simulink model "hcu_main_ADASwEPS"  (Simulink 8.2)
settings: Solver=FixedStepDiscrete  StartTime=0.0  StopTime=inf  FixedStep=0.001  RelTol=1e-3
PostLoadFcn:
  | , if any(exist('dsrtsu_mdlpostloadfcn', 'file') == [2, 3, 6]), try dsrtsu_mdlpostloadfcn('Execute', bdroot); catch fprintf('Error in PostLoadFcn (dsrtsu_mdlpostloadfcn) for model "%s":\n %s\n', bdroot, lasterr); end, end,
values from neighbouring files (symbols this model uses):
  C_TASK_1MS_S = (	C_TICK_TIME_S       )    [hcu_local_hdr.m]    (also in temp_ovrd_values.m = double(	0.001                  ))
  C_TASK_5MS_S = (	C_TICK_TIME_S      	)    [hcu_local_hdr.m]
  ENUM_ADASLFCSTATUS_OFF = uint8(  0  )    [hcu_local_hdr.m]
  ENUM_ADASLFCSTATUS_STANDBY = uint8(  1  )    [hcu_local_hdr.m]
  ENUM_ADASLKASTATUS_ACTIVE = uint8(  2  )    [hcu_local_hdr.m]
  ENUM_ADASLKASTATUS_OFF = uint8(  0  )    [hcu_local_hdr.m]
  ENUM_ADASLKASTATUS_STANDBY = uint8(  1  )    [hcu_local_hdr.m]
  ENUM_EPSMODEREQ_ANGLE = uint8(  1  )    [hcu_local_hdr.m]
  ENUM_EPSMODEREQ_INTERNAL = uint8(  0  )    [hcu_local_hdr.m]
  ENUM_EPSMODEREQ_TORQUE = uint8(  2  )    [hcu_local_hdr.m]
  ENUM_GEARPOSN_1ST = uint8(  1  )    [hcu_local_hdr.m]
  ENUM_GEARPOSN_2ND = uint8(  2  )    [hcu_local_hdr.m]
  ENUM_GEARPOSN_3RD = uint8(  3  )    [hcu_local_hdr.m]
  ENUM_GEARPOSN_4TH = uint8(  4  )    [hcu_local_hdr.m]
  ENUM_GEARPOSN_5TH = uint8(  5  )    [hcu_local_hdr.m]
  ENUM_GEARPOSN_6TH = uint8(  6  )    [hcu_local_hdr.m]
  ENUM_GEARPOSN_PN = uint8(  0  )    [hcu_local_hdr.m]
  ENUM_GEARPOSN_R = uint8(  7  )    [hcu_local_hdr.m]
  FALSE = boolean( 0 )    [hcu_local_hdr.m]
  TRUE = boolean( 1 )    [hcu_local_hdr.m]
undefined symbols (not defined in the file or in its folder): AACC_DistCtrlIMult_X_mps2, AACC_DistCtrlPMult_X_mps2, AACC_GearActual_enum, AACC_SpdCtrlIMult_X_mps2, AACC_SpdCtrlPMult_X_mps2, AACC_VehSpd_kph, AISP_EPSCurrent_pct, AISP_TqASensorDelta_pct, AISP_TqBSensorDelta_pct, ENUM_ACCSTATUS_ACTIVE, ENUM_ACCSTATUS_OFF, ENUM_ACCSTATUS_STANDBY, ENUM_ADASLFCSTATUS_ACTIVE, ENUM_ADASLFCSTATUS_TRANSITION, ENUM_LFCCCONTSTATUS_ACTIVE, ENUM_LFCCCONTSTATUS_NOTAVAIL_TEMP, ENUM_LFCCCONTSTATUS_OFF, ENUM_LFCCCONTSTATUS_READY, ENUM_LFCCCONTSTATUS_TRANSITION, ENUM_LKACCONTSTATUS_ACTIVE, ENUM_LKACCONTSTATUS_NOTAVAIL_TEMP, ENUM_LKACCONTSTATUS_OFF, ENUM_LKACCONTSTATUS_READY, KACC_AcclReqMax_g, KACC_AcclReqMin_g, KACC_ACCSetTimeGapDef1_s, KACC_ACCSetTimeGapDef2_s, KACC_ACCSetTimeGapDef3_s, KACC_ACCSetTimeGapDef4_s, KACC_ACCSetTimeGapDef5_s, KACC_AirDensity_kgpm3, KACC_AirDragCoef_rat, KACC_CommandsOn_flg, KACC_CruzSpdChgTimeThres_s, KACC_DecReqSwOffThres_Nm, KACC_DecReqSwOnThres_Nm, KACC_DistCtrlAdjTime_s, KACC_DistCtrlCalRate_s, KACC_DistCtrlIC_mps2, KACC_DistCtrlIGain_rat, KACC_DistCtrlIMax_mps2, KACC_DistCtrlIMin_mps2, KACC_DistCtrlIRest_flg, KACC_DistCtrlKGain_rat, KACC_DistCtrlPause_flg, KACC_DistCtrlPGain_rat, KACC_FinalDriveEff_pct, KACC_FinalDriveRatio_rat, KACC_FrontalArea_m2, KACC_GearBoxEff_pct, KACC_LongPushSpdChg_kph, KACC_MaxAccSetSpd_kph, KACC_MinAccSetSpd_kph, KACC_SetAllowSpdLim_kph, KACC_SpdCtrlAdjTime_s, KACC_SpdCtrlCalRate_s, KACC_SpdCtrlIC_mps2, KACC_SpdCtrlIGain_rat, KACC_SpdCtrlIMax_mps2, KACC_SpdCtrlIMin_mps2 ... (+26)
libraries: simulink x54, adas_lib x6, rti1401lib_dio_type3 x4, rtimmsu_dsrtlib x3, hcu_lib x2, aeb x1, ddm x1, dfr x1, dgi x1, dhp x1, dinr x1, dip x1
(part 7 of 9)

== system hcu_main_ADASwEPS/EPSS/EPSS/TorqueMode ==
  VISP_StrTqReq_Nm : Inport
  VISP_StrTqReqAppl_flg : Inport  Port=2
  VEPSS_StrWhlTqReqAst_Nm : Inport  Port=3
  VISP_EPSModeReq_enum : Inport  Port=4
  VISP_ADASLFCStatus_enum : Inport  Port=5
  VISP_ADASLFCMode_enum : Inport  Port=6
  Constant1 : Constant  Value=ENUM_LFCCCONTSTATUS_ACTIVE
  Constant10 : Constant  Value=ENUM_ADASLFCSTATUS_OFF
  Constant11 : Constant  Value=ENUM_LFCCCONTSTATUS_NOTAVAIL_TEMP
  Constant2 : Constant  Value=ENUM_LFCCCONTSTATUS_TRANSITION
  Constant3 : Constant  Value=ENUM_LFCCCONTSTATUS_READY
  Constant4 : Constant  Value=ENUM_ADASLFCSTATUS_TRANSITION
  Constant5 : Constant  Value=ENUM_LFCCCONTSTATUS_TRANSITION
  Constant6 : Constant  Value=ENUM_EPSMODEREQ_TORQUE
  Constant7 : Constant  Value=ENUM_ADASLFCSTATUS_ACTIVE
  Constant8 : Constant  Value=ENUM_LFCCCONTSTATUS_OFF
  Constant9 : Constant  Value=ENUM_ADASLFCSTATUS_STANDBY
  Logical Operator : Logic  Inputs=3  AllPortsSameDT=off  OutDataTypeStr=boolean
  Relational Operator{1..6} (6 alike) : RelationalOperator  Operator===  OutDataTypeStr=boolean
  Sum : Sum
  Switch{1..6} (6 alike) : Switch  Criteria=u2 ~= 0
  VEPSS_StrWhlTqReqTq_Nm : Outport
  VEPSS_TorqueModeActive_flg : Outport  Port=2
  VEPSS_LFCContStatusTq_enum : Outport  Port=3
  wires:
  Sum/1 -> Switch2/1
  VISP_StrTqReq_Nm/1 -> Switch2/3, Sum/2
  Switch4/1 -> VEPSS_StrWhlTqReqTq_Nm/1  "VEPSS_StrWhlTqReqTq_Nm"
  Constant1/1 -> Switch3/3
  Switch1/1 -> VEPSS_LFCContStatusTq_enum/1, [VEPSS_LFCContStatus_enum]  "VEPSS_LFCContStatusTq_enum"
  VEPSS_StrWhlTqReqAst_Nm/1 -> [VEPSS_StrWhlTqReqAst_Nm], Sum/1
  Switch2/1 -> Switch4/1
  VISP_ADASLFCMode_enum/1 -> Relational Operator1/1
  Constant4/1 -> Relational Operator1/2
  Switch3/1 -> Switch1/1
  Relational Operator1/1 -> Switch3/2
  Constant2/1 -> Switch3/1
  [VEPSS_TorqueModeActive_flg] -> Switch4/2
  [VEPSS_LFCContStatus_enum] -> Relational Operator2/1
  Constant5/1 -> Relational Operator2/2
  Relational Operator2/1 -> Switch2/2
  [VEPSS_StrWhlTqReqAst_Nm] -> Switch4/3
  [VEPSS_TorqueModeActive_flg] -> VEPSS_TorqueModeActive_flg/1  "VEPSS_TorqueModeActive_flg"
  VISP_EPSModeReq_enum/1 -> Relational Operator3/1
  Constant6/1 -> Relational Operator3/2
  VISP_StrTqReqAppl_flg/1 -> Logical Operator/1
  Logical Operator/1 -> Switch1/2, [VEPSS_TorqueModeActive_flg]
  Relational Operator3/1 -> Logical Operator/2
  Constant7/1 -> Relational Operator4/2
  Relational Operator4/1 -> Logical Operator/3
  Switch5/1 -> Switch1/3
  Constant9/1 -> Relational Operator5/2
  Relational Operator5/1 -> Switch5/2
  Constant3/1 -> Switch5/1
  Switch6/1 -> Switch5/3
  VISP_ADASLFCStatus_enum/1 -> Relational Operator6/1, Relational Operator5/1, Relational Operator4/1
  Constant10/1 -> Relational Operator6/2
  Relational Operator6/1 -> Switch6/2
  Constant8/1 -> Switch6/1
  Constant11/1 -> Switch6/3

== system hcu_main_ADASwEPS/EPSS/model_info/EmptySubsystem ==

== system hcu_main_ADASwEPS/ISP/AngleProcessing/Timer ==
  Enable : EnablePort  StatesWhenEnabling=reset
  C_TASK_1MS_S : Constant  Value=C_TASK_1MS_S
  Sum : Sum  Inputs=|++
  Unit Delay : UnitDelay  SampleTime=-1
  Unit Delay1 : UnitDelay  SampleTime=-1
  Time_s : Outport  OutputWhenDisabled=reset  InitialOutput=[0]
  wires:
  C_TASK_1MS_S/1 -> Unit Delay1/1
  Sum/1 -> Unit Delay/1, Time_s/1  "Time_s"
  Unit Delay/1 -> Sum/2
  Unit Delay1/1 -> Sum/1

== system hcu_main_ADASwEPS/ISP/AngleProcessing/Triggered Absolute Angle Zero ==
  In : Inport
  Trigger : TriggerPort
  SteerAngValid_flg : Constant  Value=TRUE
  Out1 : Outport
  Out2 : Outport  Port=2
  wires:
  In/1 -> Out1/1
  SteerAngValid_flg/1 -> Out2/1

== system hcu_main_ADASwEPS/ISP/PassThrough/EPSDegTest ==
  PassThrough : Inport
  AmplitudeDeg_pct : Constant  Value=5
  Compare To Constant : simulink/Logic and Bit Operations/Compare To Constant  relop===  const=3.0  OutDataTypeStr=boolean
  Constant : Constant  Value=2*pi  OutDataTypeStr=single
  DegSetPt : Constant
  FrequencyDeg_Hz : Constant
  Multiport Switch1 : MultiPortSwitch  Inputs=4
  Product : Product  Inputs=3  RndMeth=Zero
  Product1 : Product  RndMeth=Zero
  TestModeDeg_Sw : Constant
  Timer : Subsystem
  Trigonometric Funcon : Trigonometry
  DegOut : Outport
  wires:
  Multiport Switch1/1 -> DegOut/1  "DegOut"
  PassThrough/1 -> Multiport Switch1/2
  DegSetPt/1 -> Multiport Switch1/3
  Product1/1 -> Multiport Switch1/4
  FrequencyDeg_Hz/1 -> Product/2
  Product/1 -> Trigonometric Funcon/1
  AmplitudeDeg_pct/1 -> Product1/2
  Trigonometric Funcon/1 -> Product1/1
  Constant/1 -> Product/3
  Timer/1(SineTime_s) -> Product/1
  TestModeDeg_Sw/1 -> Compare To Constant/1, Multiport Switch1/1
  Compare To Constant/1 -> Timer/Enable

== system hcu_main_ADASwEPS/ISP/TqProcessing/LowPassFilter ==
  Raw : Inport
  Constant1 : Constant  OutDataTypeStr=single  SampleTime=-1
  LowPassCoef : Constant  SampleTime=-1
  Product : Product  RndMeth=Zero
  Product1 : Product  RndMeth=Zero
  Sum1 : Sum  Inputs=+-
  Sum2 : Sum
  Unit Delay1 : UnitDelay  SampleTime=-1
  Out : Outport
  wires:
  Raw/1 -> Product/2
  Constant1/1 -> Sum1/1
  LowPassCoef/1 -> [LowPassCoef], Product/1
  [LowPassCoef] -> Sum1/2
  Unit Delay1/1 -> Product1/1
  Sum1/1 -> Product1/2
  Product/1 -> Sum2/1
  Product1/1 -> Sum2/2
  Sum2/1 -> Unit Delay1/1, Out/1

== system hcu_main_ADASwEPS/ISP/TqProcessing/TorqueValid ==
  TqA : Inport
  TqB : Inport  Port=2
  Abs1 : Abs
  FALSE : Constant  Value=FALSE  OutDataTypeStr=single  SampleTime=-1
  Relational Operator1 : RelationalOperator  Operator=<=  OutDataTypeStr=boolean
  Sum1 : Sum  Inputs=+-
  Switch1 : Switch  Criteria=u2 ~= 0
  TRUE : Constant  Value=TRUE  OutDataTypeStr=single  SampleTime=-1
  TqValidThres_Nm : Constant  OutDataTypeStr=single  SampleTime=-1
  TqValid_flg : Outport
  wires:
  TRUE/1 -> Switch1/1
  TqValidThres_Nm/1 -> Relational Operator1/2
  Relational Operator1/1 -> Switch1/2
  Sum1/1 -> Abs1/1
  Abs1/1 -> Relational Operator1/1
  FALSE/1 -> Switch1/3
  Switch1/1 -> TqValid_flg/1  "TqValid_flg"
  TqA/1 -> Sum1/1
  TqB/1 -> Sum1/2

== system hcu_main_ADASwEPS/ISP/TqProcessing/TqSensorAZero ==
  VHAL_TqSensorADuty_pct : Inport
  TqSensorFlac_pct : Inport  Port=2
  KISP_EPSZeroReset_flg : Inport  Port=3
  Constant1 : Constant  Value=60  OutDataTypeStr=single  SampleTime=-1
  Constant2 : Constant  Value=50  OutDataTypeStr=single  SampleTime=-1
  Delay : Delay  DelayLength=1  InitialCondition=0
  Delay1 : Delay  DelayLength=1  InitialCondition=1
  Delay2 : Delay  DelayLength=1  InitialCondition=1
  FALSE : Constant  Value=FALSE
  Gain : Gain  Gain=-1
  IsInRange : adas_lib/IsInRange
  IsInRange1 : adas_lib/IsInRange
  KISP_CheckZeroTime_s : Constant  Value=3
  Latch : Subsystem
  Logical Operator : Logic  Operator=NOT  AllPortsSameDT=off  OutDataTypeStr=boolean
  Logical Operator1 : Logic  Operator=OR  AllPortsSameDT=off  OutDataTypeStr=boolean
  Logical Operator4 : Logic  AllPortsSameDT=off  OutDataTypeStr=boolean
  Relational Operator : RelationalOperator  Operator=<=  OutDataTypeStr=boolean
  Subtract : Sum  Inputs=+-
  Subtract1 : Sum  Inputs=+-
  Switch : Switch  Criteria=u2 ~= 0
  Switch1 : Switch  Criteria=u2 ~= 0
  Timer : Subsystem
  zero : Outport
  delta : Outport  Port=2
  wires:
  Relational Operator/1 -> Switch/2
  Logical Operator1/1 -> Latch/2(update)
  KISP_EPSZeroReset_flg/1 -> Logical Operator1/1
  Delay1/1 -> Logical Operator1/2
  Latch/1(out) -> Subtract/2, Switch/3
  Switch/1 -> Delay/1, Subtract1/2, zero/1
  KISP_CheckZeroTime_s/1 -> Relational Operator/2
  Timer/1(Time_s) -> Relational Operator/1
  Subtract/1 -> IsInRange/1
  VHAL_TqSensorADuty_pct/1 -> Subtract/1, IsInRange1/1, Switch1/1, Subtract1/1, Latch/1(in)
  Gain/1 -> IsInRange/3
  TqSensorFlac_pct/1 -> Gain/1, IsInRange/2
  Subtract1/1 -> delta/1
  IsInRange/1 -> Logical Operator4/2, Logical Operator/1
  Switch1/1 -> Switch/1
  Logical Operator/1 -> Delay1/1
  FALSE/1 -> Delay2/1
  Delay2/1 -> Switch1/2
  Delay/1 -> Switch1/3
  Logical Operator4/1 -> Timer/Enable
  IsInRange1/1 -> Logical Operator4/1
  Constant1/1 -> IsInRange1/2
  Constant2/1 -> IsInRange1/3

== system hcu_main_ADASwEPS/ISP/TqProcessing/TqSensorBZero ==
  VHAL_TqSensorBDuty_pct : Inport
  TqSensorFlac_pct : Inport  Port=2
  KISP_EPSZeroReset_flg : Inport  Port=3
  Constant1 : Constant  Value=60  OutDataTypeStr=single  SampleTime=-1
  Constant2 : Constant  Value=50  OutDataTypeStr=single  SampleTime=-1
  Delay : Delay  DelayLength=1  InitialCondition=0
  Delay1 : Delay  DelayLength=1  InitialCondition=1
  Delay2 : Delay  DelayLength=1  InitialCondition=1
  FALSE : Constant  Value=FALSE
  Gain : Gain  Gain=-1
  IsInRange : adas_lib/IsInRange
  IsInRange1 : adas_lib/IsInRange
  KISP_CheckZeroTime_s : Constant  Value=3
  Latch : Subsystem
  Logical Operator : Logic  Operator=NOT  AllPortsSameDT=off  OutDataTypeStr=boolean
  Logical Operator1 : Logic  Operator=OR  AllPortsSameDT=off  OutDataTypeStr=boolean
  Logical Operator4 : Logic  AllPortsSameDT=off  OutDataTypeStr=boolean
  Relational Operator : RelationalOperator  Operator=<=  OutDataTypeStr=boolean
  Subtract : Sum  Inputs=+-
  Subtract1 : Sum  Inputs=+-
  Switch : Switch  Criteria=u2 ~= 0
  Switch1 : Switch  Criteria=u2 ~= 0
  Timer : Subsystem
  zero : Outport
  delta : Outport  Port=2
  wires:
  Constant2/1 -> IsInRange1/3
  Constant1/1 -> IsInRange1/2
  IsInRange1/1 -> Logical Operator4/1
  Logical Operator4/1 -> Timer/Enable
  Delay/1 -> Switch1/3
  Delay2/1 -> Switch1/2
  FALSE/1 -> Delay2/1
  Logical Operator/1 -> Delay1/1
  Switch1/1 -> Switch/1
  IsInRange/1 -> Logical Operator/1, Logical Operator4/2
  Subtract1/1 -> delta/1
  TqSensorFlac_pct/1 -> IsInRange/2, Gain/1
  Gain/1 -> IsInRange/3
  VHAL_TqSensorBDuty_pct/1 -> Subtract/1, IsInRange1/1, Subtract1/1, Switch1/1, Latch/1(in)
  Subtract/1 -> IsInRange/1
  Timer/1(Time_s) -> Relational Operator/1
  KISP_CheckZeroTime_s/1 -> Relational Operator/2
  Switch/1 -> zero/1, Subtract1/2, Delay/1
  Latch/1(out) -> Switch/3, Subtract/2
  Delay1/1 -> Logical Operator1/2
  KISP_EPSZeroReset_flg/1 -> Logical Operator1/1
  Logical Operator1/1 -> Latch/2(update)
  Relational Operator/1 -> Switch/2

== system hcu_main_ADASwEPS/OSP/OSP/CheckSum Calculation ==
  BISP_outputs : Inport
  LifeCount : Inport  Port=2
  Byte0 : Subsystem
  Byte1 : Subsystem
  Byte2 : Subsystem
  Byte3 : Subsystem
  ChecksumCalculation : Subsystem  TreatAsAtomicUnit=on
  VOSP_SAS1CalcChecksum_raw8 : Outport
  wires:
  Byte0/2(ForByte1) -> Byte1/1(ForByte1)
  BISP_outputs/1 -> Byte0/1(BISP_outputs), Byte3/1(BISP_outputs)
  LifeCount/1 -> ChecksumCalculation/5(SAS_MsgCount)
  ChecksumCalculation/1(Message_Checksum) -> VOSP_SAS1CalcChecksum_raw8/1  "VOSP_SAS1CalcChecksum_raw8"
  Byte0/1(Byte0) -> ChecksumCalculation/1(Byte0)
  Byte1/1(Byte1) -> ChecksumCalculation/2(Byte1)
  Byte3/1(Byte3) -> ChecksumCalculation/4(Byte3)
  Byte2/1(Byte2) -> ChecksumCalculation/3(Byte2)

== system hcu_main_ADASwEPS/OSP/OSP/CheckSum Calculation1 ==
  BISP_outputs : Inport
  LifeCount : Inport  Port=2
  Byte0 : Subsystem
  Byte1 : Subsystem
  Byte2 : Subsystem
  Byte3 : Subsystem
  ChecksumCalculation : Subsystem  TreatAsAtomicUnit=on
  Terminator : Terminator
  VOSP_EPAS2CalcChecksum_raw8 : Outport
  wires:
  ChecksumCalculation/1(Message_Checksum) -> VOSP_EPAS2CalcChecksum_raw8/1  "VOSP_EPAS2CalcChecksum_raw8"
  LifeCount/1 -> ChecksumCalculation/5(EPAS2_MsgCount)
  BISP_outputs/1 -> Byte2/1(BISP_outputs), Byte3/1(BISP_outputs), Byte1/1(BISP_outputs)
  Byte0/1(Byte0) -> ChecksumCalculation/1(Byte0)
  Byte1/1(Byte1) -> ChecksumCalculation/2(Byte1)
  Byte2/1(Byte2) -> ChecksumCalculation/3(Byte2)
  Byte3/1(Byte3) -> ChecksumCalculation/4(Byte3)
  Byte3/2(ForByte4) -> Terminator/1

== system hcu_main_ADASwEPS/OSP/OSP/RollCnt ==
  max : Inport
  Add : Sum
  Constant : Constant  OutDataTypeStr=Inherit: Inherit via back propagation
  Constant1 : Constant  Value=0  OutDataTypeStr=Inherit: Inherit via back propagation
  Data Type Conversion6 : DataTypeConversion  OutDataTypeStr=uint8
  Relational Operator : RelationalOperator  Operator=>  OutDataTypeStr=boolean
  Switch2 : Switch  Criteria=u2 ~= 0
  Unit Delay1 : UnitDelay  SampleTime=-1
  out : Outport
  wires:
  Constant/1 -> Add/1
  Add/1 -> Switch2/3, Relational Operator/1
  Unit Delay1/1 -> Add/2
  Constant1/1 -> Switch2/1
  Switch2/1 -> Unit Delay1/1, Data Type Conversion6/1
  max/1 -> Relational Operator/2
  Relational Operator/1 -> Switch2/2
  Data Type Conversion6/1 -> out/1

== system hcu_main_ADASwEPS/OSP/OSP/RollCnt1 ==
  max : Inport
  Add : Sum
  Constant : Constant  OutDataTypeStr=Inherit: Inherit via back propagation
  Constant1 : Constant  Value=0  OutDataTypeStr=Inherit: Inherit via back propagation
  Data Type Conversion6 : DataTypeConversion  OutDataTypeStr=uint8
  Relational Operator : RelationalOperator  Operator=>  OutDataTypeStr=boolean
  Switch2 : Switch  Criteria=u2 ~= 0
  Unit Delay1 : UnitDelay  SampleTime=-1
  out : Outport
  wires:
  Data Type Conversion6/1 -> out/1
  Relational Operator/1 -> Switch2/2
  max/1 -> Relational Operator/2
  Switch2/1 -> Data Type Conversion6/1, Unit Delay1/1
  Constant1/1 -> Switch2/1
  Unit Delay1/1 -> Add/2
  Add/1 -> Relational Operator/1, Switch2/3
  Constant/1 -> Add/1

== system hcu_main_ADASwEPS/OSP/OSP/RollCnt2 ==
  max : Inport
  Add : Sum
  Constant : Constant  OutDataTypeStr=Inherit: Inherit via back propagation
  Constant1 : Constant  Value=0  OutDataTypeStr=Inherit: Inherit via back propagation
  Data Type Conversion6 : DataTypeConversion  OutDataTypeStr=uint8
  Relational Operator : RelationalOperator  Operator=>  OutDataTypeStr=boolean
  Switch2 : Switch  Criteria=u2 ~= 0
  Unit Delay1 : UnitDelay  SampleTime=-1
  out : Outport
  wires:
  Constant/1 -> Add/1
  Add/1 -> Switch2/3, Relational Operator/1
  Unit Delay1/1 -> Add/2
  Constant1/1 -> Switch2/1
  Switch2/1 -> Unit Delay1/1, Data Type Conversion6/1
  max/1 -> Relational Operator/2
  Relational Operator/1 -> Switch2/2
  Data Type Conversion6/1 -> out/1

== system hcu_main_ADASwEPS/RTI Data/RTI Data Store/RTI Data Store ==
  RTI Data Store : Subsystem  mask(RTI_DATA_STORE){}
      mask help:
      | RTI Data Store Block. This block is used by RTI to store internal model dependent data. Deleting this block will result in data loss.
      |
      | NEVER DELETE, COPY, OR MODIFY THIS BLOCK!
      mask Help:
      | RTI Data Store Block. This block is used by RTI to store internal model dependent data. Deleting this block will result in data loss.
      | 
      | NEVER DELETE, COPY, OR MODIFY THIS BLOCK!
      mask Display: text(0.5, 0.5, ' ', 'HorizontalAlignment', 'center');

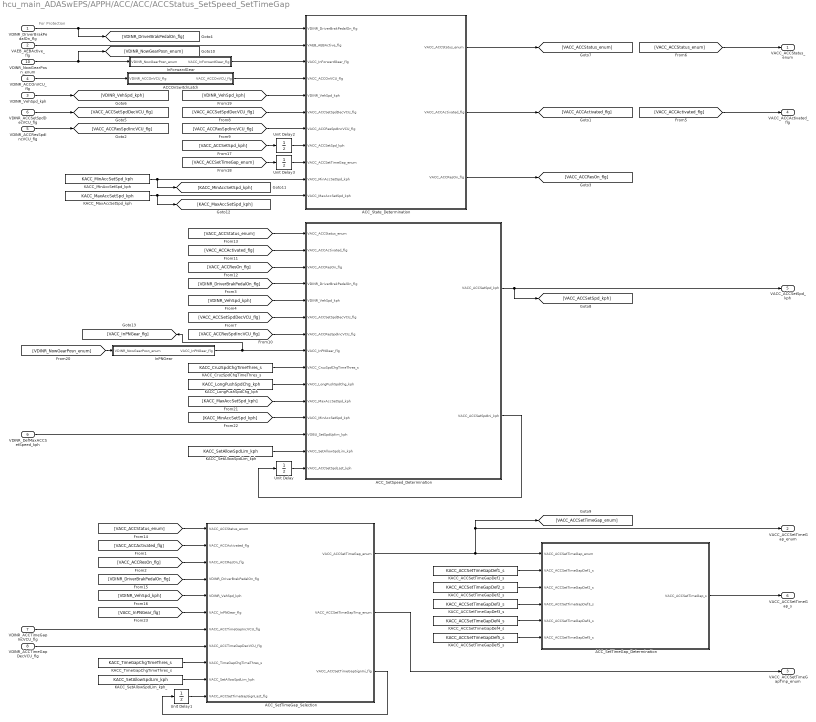
== system hcu_main_ADASwEPS/APPH/ACC/ACC/ACCStatus_SetSpeed_SetTimeGap ==
  note: For Protection
  VDINR_DriverBrakPedalOn_flg : Inport
  VAEB_AEBActive_flg : Inport  Port=2
  VDINR_VehSpd_kph : Inport  Port=3
  VDINR_ACCOnVCU_flg : Inport  Port=4
  VDINR_ACCResSpdIncVCU_flg : Inport  Port=5
  VDINR_ACCSetSpdDecVCU_flg : Inport  Port=6
  VDINR_ACCTimeGapIncVCU_flg : Inport  Port=7
  VDINR_ACCTimeGapDecVCU_flg : Inport  Port=8
  VDINR_DefMaxACCSetSpeed_kph : Inport  Port=9
  VDINR_NowGearPosn_enum : Inport  Port=10
  ACCOnSwitchLatch : Stateflow chart  TreatAsAtomicUnit=on
  ACC_SetSpeed_Determination : Stateflow chart  TreatAsAtomicUnit=on
  ACC_SetTimeGap_Determination : Stateflow chart  TreatAsAtomicUnit=on
  ACC_SetTimeGap_Selection : Stateflow chart  TreatAsAtomicUnit=on
  ACC_State_Determination : Stateflow chart  TreatAsAtomicUnit=on
  InForwardGear : Subsystem
  InPNGear : Subsystem
  KACC_ACCSetTimeGapDef1_s : Constant  Value=KACC_ACCSetTimeGapDef1_s
  KACC_ACCSetTimeGapDef2_s : Constant  Value=KACC_ACCSetTimeGapDef2_s
  KACC_ACCSetTimeGapDef3_s : Constant  Value=KACC_ACCSetTimeGapDef3_s
  KACC_ACCSetTimeGapDef4_s : Constant  Value=KACC_ACCSetTimeGapDef4_s
  KACC_ACCSetTimeGapDef5_s : Constant  Value=KACC_ACCSetTimeGapDef5_s
  KACC_CruzSpdChgTimeThres_s : Constant  Value=KACC_CruzSpdChgTimeThres_s
  KACC_LongPushSpdChg_kph : Constant  Value=KACC_LongPushSpdChg_kph
  KACC_MaxAccSetSpd_kph : Constant  Value=KACC_MaxAccSetSpd_kph
  KACC_MinAccSetSpd_kph : Constant  Value=KACC_MinAccSetSpd_kph
  KACC_SetAllowSpdLim_kph : Constant  Value=KACC_SetAllowSpdLim_kph
  KACC_SetAllowSpdLim_kph_ : Constant  Value=KACC_SetAllowSpdLim_kph
  KACC_TimeGapChgTimeThres_s : Constant  Value=KACC_TimeGapChgTimeThres_s
  Unit Delay{,1..3} (4 alike) : UnitDelay  SampleTime=-1
  VACC_ACCStatus_enum : Outport
  VACC_ACCSetTimeGap_enum : Outport  Port=2
  VACC_ACCSetTimeGapTmp_enum : Outport  Port=3
  VACC_ACCActivated_flg : Outport  Port=4
  VACC_ACCSetSpd_kph : Outport  Port=5
  VACC_ACCSetTimeGap_s : Outport  Port=6
  wires:
  KACC_CruzSpdChgTimeThres_s/1 -> ACC_SetSpeed_Determination/9(VACC_CruzSpdChgTimeThres_s)
  VDINR_ACCResSpdIncVCU_flg/1 -> [VACC_ACCResSpdIncVCU_flg]
  VDINR_ACCSetSpdDecVCU_flg/1 -> [VACC_ACCSetSpdDecVCU_flg]
  VDINR_ACCOnVCU_flg/1 -> ACCOnSwitchLatch/1(VDINR_ACCOnVCU_flg)
  ACC_SetSpeed_Determination/1(VACC_ACCSetSpd_kph) -> [VACC_ACCSetSpd_kph], VACC_ACCSetSpd_kph/1
  ACC_SetSpeed_Determination/2(VACC_ACCSetSpdIni_kph) -> Unit Delay/1
  [VDINR_VehSpd_kph] -> ACC_SetSpeed_Determination/5(VDINR_VehSpd_kph)
  [VACC_ACCResSpdIncVCU_flg] -> ACC_SetSpeed_Determination/7(VACC_ACCResSpdIncVCU_flg)
  [VACC_ACCSetSpdDecVCU_flg] -> ACC_SetSpeed_Determination/6(VACC_ACCSetSpdDecVCU_flg)
  [VACC_ACCResSpdIncVCU_flg] -> ACC_State_Determination/7(VACC_ACCResSpdIncVCU_flg)
  [VACC_ACCSetSpdDecVCU_flg] -> ACC_State_Determination/6(VACC_ACCSetSpdDecVCU_flg)
  VDINR_DriverBrakPedalOn_flg/1 -> [VDINR_DriverBrakPedalOn_flg], ACC_State_Determination/1(VDINR_DriverBrakPedalOn_flg)
  ACC_State_Determination/3(VACC_ACCResOn_flg) -> [VACC_ACCResOn_flg]
  ACC_State_Determination/2(VACC_ACCActivated_flg) -> [VACC_ACCActivated_flg]
  VDINR_VehSpd_kph/1 -> [VDINR_VehSpd_kph]
  ACCOnSwitchLatch/1(VACC_ACCOnVCU_flg) -> ACC_State_Determination/4(VACC_ACCOnVCU_flg)
  KACC_LongPushSpdChg_kph/1 -> ACC_SetSpeed_Determination/10(VACC_LongPushSpdChg_kph)
  [KACC_MinAccSetSpd_kph] -> ACC_SetSpeed_Determination/12(VACC_MinAccSetSpd_kph)
  VDINR_ACCTimeGapIncVCU_flg/1 -> ACC_SetTimeGap_Selection/7(VACC_ACCTimeGapIncVCU_flg)
  VDINR_ACCTimeGapDecVCU_flg/1 -> ACC_SetTimeGap_Selection/8(VACC_ACCTimeGapDecVCU_flg)
  [VACC_ACCActivated_flg] -> ACC_SetTimeGap_Selection/2(VACC_ACCActivated_flg)
  [VACC_ACCResOn_flg] -> ACC_SetTimeGap_Selection/3(VACC_ACCResOn_flg)
  ACC_SetTimeGap_Selection/1(VACC_ACCSetTimeGap_enum) -> [VACC_ACCSetTimeGap_enum], VACC_ACCSetTimeGap_enum/1, ACC_SetTimeGap_Determination/1(VACC_ACCSetTimeGap_enum)
  KACC_ACCSetTimeGapDef1_s/1 -> ACC_SetTimeGap_Determination/2(VACC_ACCSetTimeGapDef1_s)
  KACC_ACCSetTimeGapDef2_s/1 -> ACC_SetTimeGap_Determination/3(VACC_ACCSetTimeGapDef2_s)
  KACC_ACCSetTimeGapDef3_s/1 -> ACC_SetTimeGap_Determination/4(VACC_ACCSetTimeGapDef3_s)
  KACC_ACCSetTimeGapDef4_s/1 -> ACC_SetTimeGap_Determination/5(VACC_ACCSetTimeGapDef4_s)
  KACC_ACCSetTimeGapDef5_s/1 -> ACC_SetTimeGap_Determination/6(VACC_ACCSetTimeGapDef5_s)
  ACC_SetTimeGap_Determination/1(VACC_ACCSetTimeGap_s) -> VACC_ACCSetTimeGap_s/1
  Unit Delay/1 -> ACC_SetSpeed_Determination/15(VACC_ACCSetSpdLast_kph)
  [KACC_MaxAccSetSpd_kph] -> ACC_SetSpeed_Determination/11(VACC_MaxAccSetSpd_kph)
  [VDINR_DriverBrakPedalOn_flg] -> ACC_SetSpeed_Determination/4(VDINR_DriverBrakPedalOn_flg)
  [VACC_ACCActivated_flg] -> VACC_ACCActivated_flg/1
  ACC_State_Determination/1(VACC_ACCStatus_enum) -> [VACC_ACCStatus_enum]
  [VACC_ACCStatus_enum] -> VACC_ACCStatus_enum/1
  [VACC_ACCActivated_flg] -> ACC_SetSpeed_Determination/2(VACC_ACCActivated_flg)
  [VACC_ACCResOn_flg] -> ACC_SetSpeed_Determination/3(VACC_ACCResOn_flg)
  [VACC_ACCStatus_enum] -> ACC_SetSpeed_Determination/1(VACC_ACCStatus_enum)
  VDINR_DefMaxACCSetSpeed_kph/1 -> ACC_SetSpeed_Determination/13(VOBU_SetSpdUplim_kph)
  KACC_SetAllowSpdLim_kph/1 -> ACC_SetSpeed_Determination/14(VACC_SetAllowSpdLim_kph)
  Unit Delay1/1 -> ACC_SetTimeGap_Selection/11(VACC_ACCSetTimeGapSignLast_flg)
  ACC_SetTimeGap_Selection/3(VACC_ACCSetTimeGapSignIni_flg) -> Unit Delay1/1
  KACC_SetAllowSpdLim_kph_/1 -> ACC_SetTimeGap_Selection/10(VACC_SetAllowSpdLim_kph)
  [VACC_ACCStatus_enum] -> ACC_SetTimeGap_Selection/1(VACC_ACCStatus_enum)
  [VDINR_DriverBrakPedalOn_flg] -> ACC_SetTimeGap_Selection/4(VDINR_DriverBrakPedalOn_flg)
  [VDINR_VehSpd_kph] -> ACC_SetTimeGap_Selection/5(VDINR_VehSpd_kph)
  KACC_TimeGapChgTimeThres_s/1 -> ACC_SetTimeGap_Selection/9(VACC_TimeGapChgTimeThres_s)
  ACC_SetTimeGap_Selection/2(VACC_ACCSetTimeGapTmp_enum) -> VACC_ACCSetTimeGapTmp_enum/1
  [VACC_ACCSetSpd_kph] -> Unit Delay2/1
  Unit Delay2/1 -> ACC_State_Determination/8(VACC_ACCSetSpd_kph)
  Unit Delay3/1 -> ACC_State_Determination/9(VACC_ACCSetTimeGap_enum)
  [VACC_ACCSetTimeGap_enum] -> Unit Delay3/1
  VAEB_AEBActive_flg/1 -> ACC_State_Determination/2(VAEB_AEBActive_flg)
  [VDINR_VehSpd_kph] -> ACC_State_Determination/5(VDINR_VehSpd_kph)
  KACC_MinAccSetSpd_kph/1 -> [KACC_MinAccSetSpd_kph], ACC_State_Determination/10(VACC_MinAccSetSpd_kph)
  KACC_MaxAccSetSpd_kph/1 -> [KACC_MaxAccSetSpd_kph], ACC_State_Determination/11(VACC_MaxAccSetSpd_kph)
  InForwardGear/1(VACC_InForwardGear_flg) -> ACC_State_Determination/3(VACC_InForwardGear_flg)
  VDINR_NowGearPosn_enum/1 -> [VDINR_NowGearPosn_enum], InForwardGear/1(VDINR_NowGearPosn_enum)
  [VDINR_NowGearPosn_enum] -> InPNGear/1(VDINR_NowGearPosn_enum)
  InPNGear/1(VACC_InPNGear_flg) -> [VACC_InPNGear_flg], ACC_SetSpeed_Determination/8(VACC_InPNGear_flg)
  [VACC_InPNGear_flg] -> ACC_SetTimeGap_Selection/6(VACC_InPNGear_flg)

== system hcu_main_ADASwEPS/APPH/ACC/ACC/ACCStrategy ==
  VACC_ACCSetSpd_kph : Inport
  VACC_ACCSetTimeGap_s : Inport  Port=2
  VDINR_VehSpd_kph : Inport  Port=3
  VMCT_MCTPositionX_m : Inport  Port=4
  VMCT_MCTRelVelocityX_mps : Inport  Port=5
  VDINR_NowGearPosn_enum : Inport  Port=6
  VDINR_EngSpd_rpm : Inport  Port=7
  VMCT_MCTInPath_flg : Inport  Port=8
  Enable : EnablePort  StatesWhenEnabling=reset
  Constant1 : Constant  Value=KACC_AcclReqMin_g
  Constant2 : Constant  Value=single(2)
  Constant3 : Constant  Value=KACC_AcclReqMax_g
  Constant9 : Constant  Value=single(0)
  Detect Decrease : simulink/Logic and Bit Operations/Detect Decrease  vinit=0.0  InputProcessing=Inherited  OutDataTypeStr=boolean
  Distance Control : Subsystem
  Gain : Gain  Gain=9.81
  Gain1 : Gain  Gain=9.81
  Limit : hcu_lib/Limit
  MinMax : MinMax  Inputs=2
  Relational Operator : RelationalOperator  Operator=>  OutDataTypeStr=boolean
  SR-Latch : hcu_lib/SR-Latch
  Speed Control : Subsystem
  Switch : Switch  Criteria=u2 ~= 0
  Timer : Subsystem
  Torque Estimation : Subsystem
  Trigger signal generator : Subsystem  TreatAsAtomicUnit=on
  Unit Delay1 : UnitDelay  SampleTime=-1
  Vehicle Acceleration Calculation : Subsystem
  VACC_TqReqRaw_Nm : Outport  OutputWhenDisabled=reset  InitialOutput=[0]
  VACC_AcclReqFinal_mps2 : Outport  Port=2  OutputWhenDisabled=reset  InitialOutput=[0]
  wires:
  Speed Control/1(VACC_SpdCtrlAcclReq_mps2) -> MinMax/1
  Limit/1 -> VACC_AcclReqFinal_mps2/1, Torque Estimation/1(VACC_AcclReqFinal_mps2)  "VACC_AcclReqFinal_mps2"
  Trigger signal generator/1(Trigger_signal) -> Vehicle Acceleration Calculation/Trigger
  VDINR_VehSpd_kph/1 -> [VDINR_VehSpd_kph]
  [VDINR_VehSpd_kph] -> Vehicle Acceleration Calculation/1(In1)
  [VDINR_VehSpd_kph] -> Speed Control/2(VDINR_VehSpd_kph)
  [VDINR_VehSpd_kph] -> Distance Control/2(VDINR_VehSpd_kph)
  Distance Control/1(VACC_DistCtrlAcclReq_mps2) -> MinMax/2
  VACC_ACCSetTimeGap_s/1 -> Distance Control/3(VACC_ACCSetTimeGap_s)
  VACC_ACCSetSpd_kph/1 -> Speed Control/1(VACC_ACCSetSpd_kph)
  [VDINR_VehSpd_kph] -> Torque Estimation/2(VDINR_VehSpd_kph)
  Torque Estimation/1(VACC_TqReqRaw_Nm) -> VACC_TqReqRaw_Nm/1
  VDINR_EngSpd_rpm/1 -> Torque Estimation/4(VDINR_EngSpd_rpm)
  VDINR_NowGearPosn_enum/1 -> Torque Estimation/3(VDINR_NowGearPosn_enum)
  Vehicle Acceleration Calculation/1(VACC_VehAccl_mps2) -> [VACC_VehAccl_mps2]
  [VACC_VehAccl_mps2] -> Speed Control/3(VACC_VehAccl_mps2)
  [VACC_VehAccl_mps2] -> Distance Control/1(VACC_VehAccl_mps2)
  Constant3/1 -> Gain/1
  Constant1/1 -> Gain1/1
  Gain/1 -> Limit/2
  Gain1/1 -> Limit/3
  VMCT_MCTPositionX_m/1 -> Distance Control/4(VMCT_MCTPositionX_m)
  VMCT_MCTRelVelocityX_mps/1 -> Distance Control/5(VMCT_MCTRelVelocityX_mps)
  VMCT_MCTInPath_flg/1 -> [VMCT_MCTInPath_flg]
  [VMCT_MCTInPath_flg] -> Detect Decrease/1
  Detect Decrease/1 -> SR-Latch/1
  SR-Latch/1 -> Switch/2, Timer/Enable
  Timer/1(SineTime_s) -> Relational Operator/1
  Relational Operator/1 -> Unit Delay1/1
  Unit Delay1/1 -> SR-Latch/2
  Constant2/1 -> Relational Operator/2
  Switch/1 -> Limit/1
  MinMax/1 -> Switch/3
  Constant9/1 -> Switch/1

== system hcu_main_ADASwEPS/APPH/ACC/ACC/CommandDetermination ==
  VACC_ACCActivated_flg : Inport
  VACC_TqReqRaw_Nm : Inport  Port=2
  VACC_AcclReq_mps2 : Inport  Port=3
  Abs : Abs
  Constant : Constant  Value=single(0)
  Constant5 : Constant  Value=single(0)
  Hysteresis (higher limit) : Subsystem  TreatAsAtomicUnit=on
  Hysteresis (lower limit) : Subsystem  TreatAsAtomicUnit=on
  KACC_CommandsOn_flg : Constant  Value=KACC_CommandsOn_flg
  KACC_DecReqSwOffThres_Nm : Constant  Value=KACC_DecReqSwOffThres_Nm
  KACC_DecReqSwOnThres_Nm : Constant  Value=KACC_DecReqSwOnThres_Nm
  KACC_TqReqSwOffThres_Nm : Constant  Value=KACC_TqReqSwOffThres_Nm
  KACC_TqReqSwOnThres_Nm : Constant  Value=KACC_TqReqSwOnThres_Nm
  Logical Operator : Logic  Inputs=3  AllPortsSameDT=off  OutDataTypeStr=boolean
  Logical Operator1 : Logic  Inputs=3  AllPortsSameDT=off  OutDataTypeStr=boolean
  Switch : Switch  Criteria=u2 ~= 0
  Switch1 : Switch  Criteria=u2 ~= 0
  VACC_TqReq_Nm : Outport
  VACC_TqReqAppl_flg : Outport  Port=2
  VACC_DecReq_mps2 : Outport  Port=3
  VACC_DecReqAppl_flg : Outport  Port=4
  wires:
  VACC_TqReqRaw_Nm/1 -> Switch/1, Hysteresis (lower limit)/1(Input), Hysteresis (higher limit)/1(Input)
  KACC_TqReqSwOnThres_Nm/1 -> Hysteresis (higher limit)/2(Switch_on_point)
  KACC_TqReqSwOffThres_Nm/1 -> Hysteresis (higher limit)/3(Switch_off_point)
  KACC_DecReqSwOnThres_Nm/1 -> Hysteresis (lower limit)/2(Switch_on_point)
  KACC_DecReqSwOffThres_Nm/1 -> Hysteresis (lower limit)/3(Switch_off_point)
  Constant/1 -> Switch/3
  Switch/1 -> VACC_TqReq_Nm/1  "VACC_TqReq_Nm"
  Hysteresis (higher limit)/1(Output) -> Logical Operator/2
  VACC_ACCActivated_flg/1 -> Logical Operator1/1, Logical Operator/1
  Logical Operator1/1 -> VACC_DecReqAppl_flg/1, Switch1/2  "VACC_DecReqAppl_flg"
  Constant5/1 -> Switch1/3
  Hysteresis (lower limit)/1(Output) -> Logical Operator1/2
  VACC_AcclReq_mps2/1 -> Switch1/1
  Switch1/1 -> Abs/1
  Abs/1 -> VACC_DecReq_mps2/1  "VACC_DecReq_mps2"
  Logical Operator/1 -> VACC_TqReqAppl_flg/1, Switch/2  "VACC_TqReqAppl_flg"
  KACC_CommandsOn_flg/1 -> Logical Operator1/3, Logical Operator/3

== system hcu_main_ADASwEPS/APPH/ACC/model_info/EmptySubsystem ==

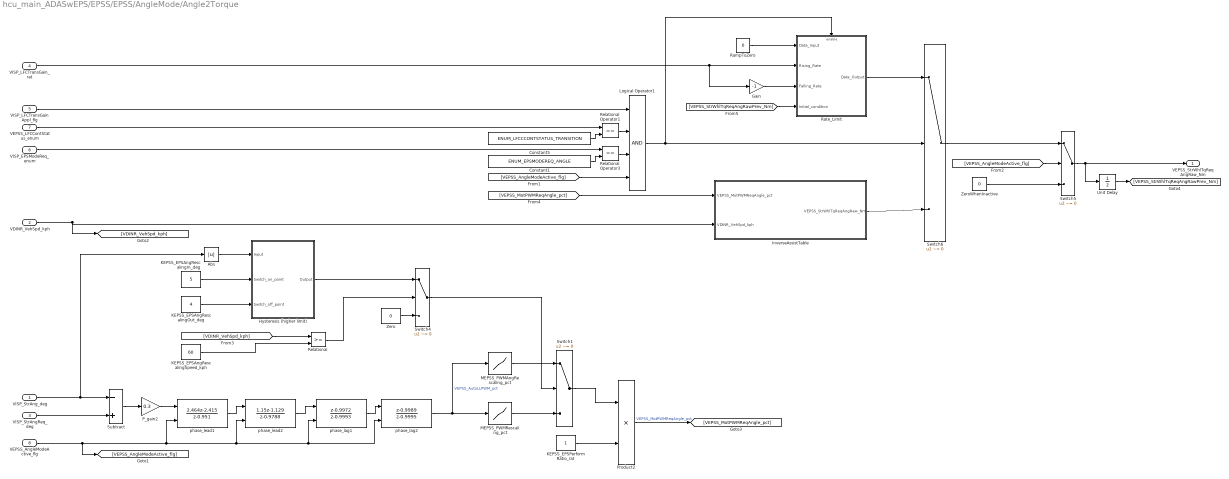
== system hcu_main_ADASwEPS/EPSS/EPSS/AngleMode/Angle2Torque ==
  VISP_StrAng_deg : Inport
  VDINR_VehSpd_kph : Inport  Port=2
  VISP_StrAngReq_deg : Inport  Port=3
  VISP_LFCTransGain_rat : Inport  Port=4
  VISP_LFCTransGainAppl_flg : Inport  Port=5
  VISP_EPSModeReq_enum : Inport  Port=6
  VEPSS_LFCContStatus_enum : Inport  Port=7
  VEPSS_AngleModeActive_flg : Inport  Port=8
  Abs : Abs
  Constant1 : Constant  Value=ENUM_EPSMODEREQ_ANGLE
  Constant5 : Constant  Value=ENUM_LFCCCONTSTATUS_TRANSITION
  Gain : Gain  Gain=-1
  Hysteresis (higher limit) : Subsystem  TreatAsAtomicUnit=on
  InverseAssistTable : Subsystem
  KEPSS_EPSAngRescalingIn_deg : Constant  Value=5  SampleTime=-1
  KEPSS_EPSAngRescalingOut_deg : Constant  Value=4  SampleTime=-1
  KEPSS_EPSAngRescalingSpeed_kph : Constant  Value=60  SampleTime=-1
  KEPSS_EPSPerformRatio_rat : Constant  SampleTime=-1
  Logical Operator1 : Logic  Inputs=4  AllPortsSameDT=off  OutDataTypeStr=boolean
  MEPSS_PWMAngRescaling_pct : Lookup  InputValues=[-100 -0.1 0 0.1 100]  Table=[-100 -0.1 0 0.1 100]  LookUpMeth=Interpolation-Use End Values
      settings: AttributesFormatString="Input=\"%<InputValues>\"\\nOutput=\"%<Table>\""
  MEPSS_PWMRescaling_pct : Lookup  InputValues=[-100 -0.1 0 0.1 100]  Table=[-100 -2.2 0 2.6 100]  LookUpMeth=Interpolation-Use End Values
      settings: AttributesFormatString="Input=\"%<InputValues>\"\\nOutput=\"%<Table>\""
  P_gain2 : Gain  Gain=0.3
  Product2 : Product  RndMeth=Zero
  RampToZero : Constant  Value=0
  Rate_Limit : Subsystem  TreatAsAtomicUnit=on
  "Relational " : RelationalOperator  OutDataTypeStr=boolean
  Relational Operator1 : RelationalOperator  Operator===  OutDataTypeStr=boolean
  Relational Operator3 : RelationalOperator  Operator===  OutDataTypeStr=boolean
  Subtract : Sum  Inputs=-+
  Switch{1,4..6} (4 alike) : Switch  Criteria=u2 ~= 0
  Unit Delay : UnitDelay  SampleTime=-1
  Zero : Constant  Value=0  SampleTime=-1
  ZeroWhenInactive : Constant  Value=0
  phase_lag1 : DiscreteTransferFcn  Numerator=[1 -0.9972]  Denominator=[1 -0.9993]  ExternalReset=Rising
      settings: InputPortMap=u0,r7
  phase_lag2 : DiscreteTransferFcn  Numerator=[1 -0.9989]  Denominator=[1 -0.9995]  ExternalReset=Rising
      settings: InputPortMap=u0,r7
  phase_lead1 : DiscreteTransferFcn  Numerator=[2.464 -2.415]  Denominator=[1 -0.951]  ExternalReset=Rising
      settings: InputPortMap=u0,r7
  phase_lead2 : DiscreteTransferFcn  Numerator=[1.15 -1.129]  Denominator=[1 -0.9788]  ExternalReset=Rising
      settings: InputPortMap=u0,r7
  VEPSS_StrWhlTqReqAngRaw_Nm : Outport
  wires:
  phase_lag2/1 -> MEPSS_PWMRescaling_pct/1, MEPSS_PWMAngRescaling_pct/1  "VEPSS_AutoLLPWM_pct"
  VISP_StrAng_deg/1 -> Subtract/1, Abs/1
  KEPSS_EPSPerformRatio_rat/1 -> Product2/2
  VISP_StrAngReq_deg/1 -> Subtract/2
  MEPSS_PWMRescaling_pct/1 -> Switch1/3
  Product2/1 -> [VEPSS_MotPWMReqAngle_pct]  "VEPSS_MotPWMReqAngle_pct"
  Subtract/1 -> P_gain2/1
  P_gain2/1 -> phase_lead1/1
  phase_lead1/1 -> phase_lead2/1
  phase_lag1/1 -> phase_lag2/1
  phase_lead2/1 -> phase_lag1/1
  MEPSS_PWMAngRescaling_pct/1 -> Switch1/1
  Switch1/1 -> Product2/1
  Switch4/1 -> Switch1/2
  KEPSS_EPSAngRescalingSpeed_kph/1 -> "Relational "/2
  "Relational "/1 -> Switch4/2
  Zero/1 -> Switch4/3
  VEPSS_LFCContStatus_enum/1 -> Relational Operator1/1
  Constant5/1 -> Relational Operator1/2
  VISP_LFCTransGainAppl_flg/1 -> Logical Operator1/1
  Relational Operator1/1 -> Logical Operator1/2
  VEPSS_AngleModeActive_flg/1 -> phase_lead2/2, phase_lag2/2, phase_lag1/2, phase_lead1/2, [VEPSS_AngleModeActive_flg]
  VISP_EPSModeReq_enum/1 -> Relational Operator3/1
  Constant1/1 -> Relational Operator3/2
  Relational Operator3/1 -> Logical Operator1/3
  InverseAssistTable/1(VEPSS_StrWhlTqReqAngRaw_Nm) -> Switch6/3
  Rate_Limit/1(Data_Output) -> Switch6/1
  RampToZero/1 -> Rate_Limit/1(Data_Input)
  Unit Delay/1 -> [VEPSS_StrWhlTqReqAngRawPrev_Nm]
  [VEPSS_StrWhlTqReqAngRawPrev_Nm] -> Rate_Limit/4(Initial_condition)
  Logical Operator1/1 -> Switch6/2, Rate_Limit/Enable
  VISP_LFCTransGain_rat/1 -> Rate_Limit/2(Rising_Rate), Gain/1
  Gain/1 -> Rate_Limit/3(Falling_Rate)
  [VEPSS_AngleModeActive_flg] -> Logical Operator1/4
  Switch6/1 -> Switch5/1
  Switch5/1 -> Unit Delay/1, VEPSS_StrWhlTqReqAngRaw_Nm/1
  [VEPSS_AngleModeActive_flg] -> Switch5/2
  ZeroWhenInactive/1 -> Switch5/3
  VDINR_VehSpd_kph/1 -> [VDINR_VehSpd_kph], InverseAssistTable/2(VDINR_VehSpd_kph)
  [VDINR_VehSpd_kph] -> "Relational "/1
  Abs/1 -> Hysteresis (higher limit)/1(Input)
  KEPSS_EPSAngRescalingIn_deg/1 -> Hysteresis (higher limit)/2(Switch_on_point)
  KEPSS_EPSAngRescalingOut_deg/1 -> Hysteresis (higher limit)/3(Switch_off_point)
  Hysteresis (higher limit)/1(Output) -> Switch4/1
  [VEPSS_MotPWMReqAngle_pct] -> InverseAssistTable/1(VEPSS_MotPWMReqAngle_pct)

== system hcu_main_ADASwEPS/EPSS/EPSS/EPSMotorPWMRequest/MotorPWMRequestCalculation ==
  VEPSS_EPSMotTqReqRaw_Nm : Inport
  1/KEPSS_PWM2TqGain_rat : Gain  Gain=0.09
  VEPSS_EPSMotPWMReqRaw_pct : Outport
  wires:
  1/KEPSS_PWM2TqGain_rat/1 -> VEPSS_EPSMotPWMReqRaw_pct/1  "VEPSS_EPSMotPWMReqRaw_pct"
  VEPSS_EPSMotTqReqRaw_Nm/1 -> 1/KEPSS_PWM2TqGain_rat/1

== system hcu_main_ADASwEPS/EPSS/EPSS/EPSMotorPWMRequest/MotorTorqueRequestCalculation ==
  VEPSS_StrWhlTqReqAst_Nm : Inport
  VEPSS_StrWhlTqReqTq_Nm : Inport  Port=2
  VEPSS_StrWhlTqReqAng_Nm : Inport  Port=3
  VEPSS_TorqueModeActive_flg : Inport  Port=4
  VEPSS_AngleModeActive_flg : Inport  Port=5
  VISP_VehSpd_kph : Inport  Port=6
  VISP_LFCTransGain_rat : Inport  Port=7
  VISP_LFCTransGainAppl_flg : Inport  Port=8
  VEPSS_LFCContStatus_enum : Inport  Port=9
  VISP_EPSModeReq_enum : Inport  Port=10
  Constant : Constant  Value=ENUM_LFCCCONTSTATUS_TRANSITION
  Constant1 : Constant  Value=ENUM_EPSMODEREQ_TORQUE
  EPSGainDefault : Constant
  KEPSS_PWM2TqGain_rat : Gain  Gain=11.1111
  Logical Operator : Logic  Operator=OR  AllPortsSameDT=off  OutDataTypeStr=boolean
  Logical Operator1 : Logic  Inputs=4  AllPortsSameDT=off  OutDataTypeStr=boolean
  MEPSS_MotorPWMRescaling_pct : Lookup  InputValues=[-100 -3 0 3 100]  Table=[-250 -3 0 3 250]  LookUpMeth=Interpolation-Use End Values
      settings: AttributesFormatString="Input=\"%<InputValues>\"\\nOutput=\"%<Table>\""
  MEPSS_TqPWMMult_rat : Lookup  InputValues=[-100 -80 -60 -40 -20 -10 0 10 20 40 60 80 100]  Table=[1 1 1 1 1 1 1 1 1 1 1 1 1]  LookUpMeth=Interpolation-Use End Values
      settings: AttributesFormatString="Input=\"%<InputValues>\"\\nOutput=\"%<Table>\""
  MEPSS_TqPWM_pct : Lookup  InputValues=[-10:0.5:10]  Table=[-20 -19 -18 -17 -16 -15 -14 -13 -12 -11 -10 -9 -8 -7 -6 -5 -4 -3 -2 -1 0 1 2 3 4 5 6 7 8 9 10 11 12 13 14 15 16 17 18 19 20]  LookUpMeth=Interpolation-Use End Values
      settings: AttributesFormatString="Input=\"%<InputValues>\"\\nOutput=\"%<Table>\""
  Product1 : Product  Inputs=3
  Relational Operator : RelationalOperator  Operator===  OutDataTypeStr=boolean
  Relational Operator1 : RelationalOperator  Operator===  OutDataTypeStr=boolean
  Switch : Switch  Criteria=u2 ~= 0
  Switch1 : Switch  Criteria=u2 ~= 0
  Switch2 : Switch  Criteria=u2 ~= 0
  VEPSS_EPSMotTqReq_Nm : Outport
  wires:
  MEPSS_TqPWMMult_rat/1 -> Product1/2
  MEPSS_TqPWM_pct/1 -> Product1/1
  VISP_VehSpd_kph/1 -> MEPSS_TqPWMMult_rat/1
  Product1/1 -> MEPSS_MotorPWMRescaling_pct/1
  VEPSS_AngleModeActive_flg/1 -> [VEPSS_AngleModeActive_flg], Switch/2
  VEPSS_StrWhlTqReqAng_Nm/1 -> Switch/1
  Switch1/1 -> Switch/3
  VEPSS_TorqueModeActive_flg/1 -> [VEPSS_TorqueModeActive_flg], Switch1/2
  VEPSS_StrWhlTqReqTq_Nm/1 -> Switch1/1
  VEPSS_StrWhlTqReqAst_Nm/1 -> Switch1/3
  Switch/1 -> MEPSS_TqPWM_pct/1
  VEPSS_LFCContStatus_enum/1 -> Relational Operator/1
  Constant/1 -> Relational Operator/2
  [VEPSS_AngleModeActive_flg] -> Logical Operator/1
  [VEPSS_TorqueModeActive_flg] -> Logical Operator/2
  VISP_LFCTransGainAppl_flg/1 -> Logical Operator1/1
  Relational Operator/1 -> Logical Operator1/2
  Logical Operator/1 -> Logical Operator1/4
  Logical Operator1/1 -> Switch2/2
  Switch2/1 -> Product1/3  "VEPSS_MotTqGain_rat"
  VISP_LFCTransGain_rat/1 -> Switch2/1
  EPSGainDefault/1 -> Switch2/3
  MEPSS_MotorPWMRescaling_pct/1 -> KEPSS_PWM2TqGain_rat/1
  KEPSS_PWM2TqGain_rat/1 -> VEPSS_EPSMotTqReq_Nm/1  "VEPSS_EPSMotTqReq_Nm"
  VISP_EPSModeReq_enum/1 -> Relational Operator1/1
  Constant1/1 -> Relational Operator1/2
  Relational Operator1/1 -> Logical Operator1/3

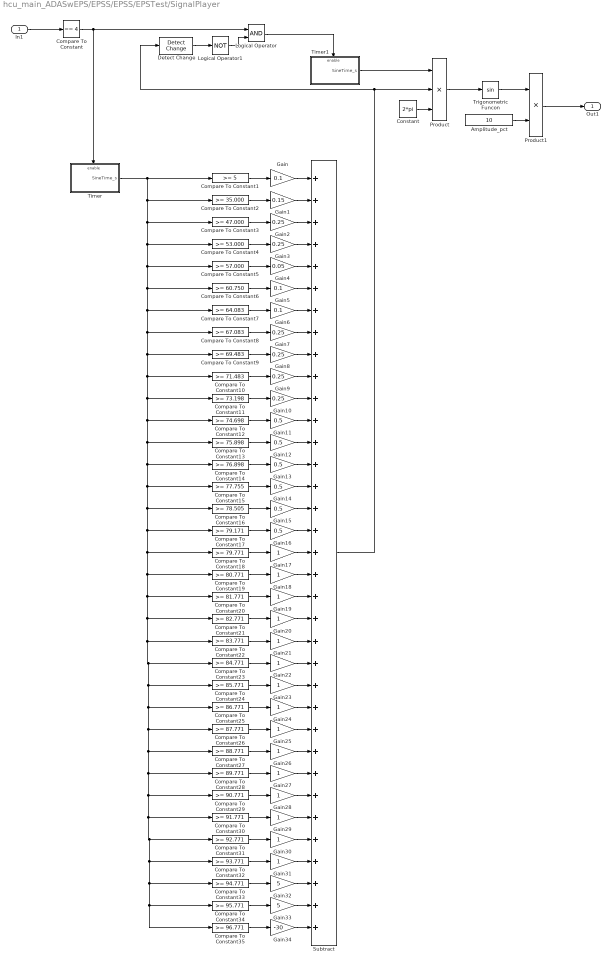
== system hcu_main_ADASwEPS/EPSS/EPSS/EPSTest/SignalPlayer ==
  In1 : Inport
  Amplitude_pct : Constant  Value=10
  Compare To Constant : simulink/Logic and Bit Operations/Compare To Constant  relop===  const=4  OutDataTypeStr=boolean
  Compare To Constant1 : simulink/Logic and Bit Operations/Compare To Constant  relop=>=  const=5  OutDataTypeStr=boolean
  Compare To Constant10 : simulink/Logic and Bit Operations/Compare To Constant  relop=>=  const=71.483  OutDataTypeStr=boolean
  Compare To Constant11 : simulink/Logic and Bit Operations/Compare To Constant  relop=>=  const=73.198  OutDataTypeStr=boolean
  Compare To Constant12 : simulink/Logic and Bit Operations/Compare To Constant  relop=>=  const=74.698  OutDataTypeStr=boolean
  Compare To Constant13 : simulink/Logic and Bit Operations/Compare To Constant  relop=>=  const=75.898  OutDataTypeStr=boolean
  Compare To Constant14 : simulink/Logic and Bit Operations/Compare To Constant  relop=>=  const=76.898  OutDataTypeStr=boolean
  Compare To Constant15 : simulink/Logic and Bit Operations/Compare To Constant  relop=>=  const=77.755  OutDataTypeStr=boolean
  Compare To Constant16 : simulink/Logic and Bit Operations/Compare To Constant  relop=>=  const=78.505  OutDataTypeStr=boolean
  Compare To Constant17 : simulink/Logic and Bit Operations/Compare To Constant  relop=>=  const=79.171  OutDataTypeStr=boolean
  Compare To Constant18 : simulink/Logic and Bit Operations/Compare To Constant  relop=>=  const=79.771  OutDataTypeStr=boolean
  Compare To Constant19 : simulink/Logic and Bit Operations/Compare To Constant  relop=>=  const=80.771  OutDataTypeStr=boolean
  Compare To Constant2 : simulink/Logic and Bit Operations/Compare To Constant  relop=>=  const=35.000  OutDataTypeStr=boolean
  Compare To Constant20 : simulink/Logic and Bit Operations/Compare To Constant  relop=>=  const=81.771  OutDataTypeStr=boolean
  Compare To Constant21 : simulink/Logic and Bit Operations/Compare To Constant  relop=>=  const=82.771  OutDataTypeStr=boolean
  Compare To Constant22 : simulink/Logic and Bit Operations/Compare To Constant  relop=>=  const=83.771  OutDataTypeStr=boolean
  Compare To Constant23 : simulink/Logic and Bit Operations/Compare To Constant  relop=>=  const=84.771  OutDataTypeStr=boolean
  Compare To Constant24 : simulink/Logic and Bit Operations/Compare To Constant  relop=>=  const=85.771  OutDataTypeStr=boolean
  Compare To Constant25 : simulink/Logic and Bit Operations/Compare To Constant  relop=>=  const=86.771  OutDataTypeStr=boolean
  Compare To Constant26 : simulink/Logic and Bit Operations/Compare To Constant  relop=>=  const=87.771  OutDataTypeStr=boolean
  Compare To Constant27 : simulink/Logic and Bit Operations/Compare To Constant  relop=>=  const=88.771  OutDataTypeStr=boolean
  Compare To Constant28 : simulink/Logic and Bit Operations/Compare To Constant  relop=>=  const=89.771  OutDataTypeStr=boolean
  Compare To Constant29 : simulink/Logic and Bit Operations/Compare To Constant  relop=>=  const=90.771  OutDataTypeStr=boolean
  Compare To Constant3 : simulink/Logic and Bit Operations/Compare To Constant  relop=>=  const=47.000  OutDataTypeStr=boolean
  Compare To Constant30 : simulink/Logic and Bit Operations/Compare To Constant  relop=>=  const=91.771  OutDataTypeStr=boolean
  Compare To Constant31 : simulink/Logic and Bit Operations/Compare To Constant  relop=>=  const=92.771  OutDataTypeStr=boolean
  Compare To Constant32 : simulink/Logic and Bit Operations/Compare To Constant  relop=>=  const=93.771  OutDataTypeStr=boolean
  Compare To Constant33 : simulink/Logic and Bit Operations/Compare To Constant  relop=>=  const=94.771  OutDataTypeStr=boolean
  Compare To Constant34 : simulink/Logic and Bit Operations/Compare To Constant  relop=>=  const=95.771  OutDataTypeStr=boolean
  Compare To Constant35 : simulink/Logic and Bit Operations/Compare To Constant  relop=>=  const=96.771  OutDataTypeStr=boolean
  Compare To Constant4 : simulink/Logic and Bit Operations/Compare To Constant  relop=>=  const=53.000  OutDataTypeStr=boolean
  Compare To Constant5 : simulink/Logic and Bit Operations/Compare To Constant  relop=>=  const=57.000  OutDataTypeStr=boolean
  Compare To Constant6 : simulink/Logic and Bit Operations/Compare To Constant  relop=>=  const=60.750  OutDataTypeStr=boolean
  Compare To Constant7 : simulink/Logic and Bit Operations/Compare To Constant  relop=>=  const=64.083  OutDataTypeStr=boolean
  Compare To Constant8 : simulink/Logic and Bit Operations/Compare To Constant  relop=>=  const=67.083  OutDataTypeStr=boolean
  Compare To Constant9 : simulink/Logic and Bit Operations/Compare To Constant  relop=>=  const=69.483  OutDataTypeStr=boolean
  Constant : Constant  Value=2*pi  OutDataTypeStr=single
  Detect Change : simulink/Logic and Bit Operations/Detect Change  vinit=0  InputProcessing=Inherited  OutDataTypeStr=boolean
  Gain : Gain  Gain=0.1
  Gain1 : Gain  Gain=0.15
  Gain{2..3,7..10} (6 alike) : Gain  Gain=0.25
  Gain{11..16} (6 alike) : Gain  Gain=0.5
  Gain{17..31} (15 alike) : Gain
  Gain32 : Gain  Gain=5
  Gain33 : Gain  Gain=5
  Gain34 : Gain  Gain=-30
  Gain4 : Gain  Gain=0.05
  Gain5 : Gain  Gain=0.1
  Gain6 : Gain  Gain=0.1
  Logical Operator : Logic  AllPortsSameDT=off  OutDataTypeStr=boolean
  Logical Operator1 : Logic  Operator=NOT  AllPortsSameDT=off  OutDataTypeStr=boolean
  Product : Product  Inputs=3  RndMeth=Zero
  Product1 : Product  RndMeth=Zero
  Subtract : Sum  Inputs=35
  Timer : Subsystem
  Timer1 : Subsystem
  Trigonometric Funcon : Trigonometry
  Out1 : Outport
  wires:
  Subtract/1 -> Product/2, Detect Change/1
  Product/1 -> Trigonometric Funcon/1
  Amplitude_pct/1 -> Product1/2
  Trigonometric Funcon/1 -> Product1/1
  Constant/1 -> Product/3
  Compare To Constant/1 -> Logical Operator/1, Timer/Enable
  In1/1 -> Compare To Constant/1
  Timer/1(SineTime_s) -> Compare To Constant2/1, Compare To Constant8/1, Compare To Constant35/1, Compare To Constant34/1, Compare To Constant33/1, Compare To Constant32/1, Compare To Constant31/1, Compare To Constant30/1, Compare To Constant29/1, Compare To Constant28/1, Compare To Constant27/1, Compare To Constant26/1, Compare To Constant25/1, Compare To Constant24/1, Compare To Constant23/1, Compare To Constant22/1, Compare To Constant21/1, Compare To Constant20/1, Compare To Constant19/1, Compare To Constant18/1, Compare To Constant17/1, Compare To Constant16/1, Compare To Constant15/1, Compare To Constant14/1, Compare To Constant13/1, Compare To Constant12/1, Compare To Constant11/1, Compare To Constant10/1, Compare To Constant9/1, Compare To Constant7/1, Compare To Constant6/1, Compare To Constant5/1, Compare To Constant4/1, Compare To Constant3/1, Compare To Constant1/1
  Compare To Constant1/1 -> Gain/1
  Gain/1 -> Subtract/1
  Compare To Constant2/1 -> Gain1/1
  Gain1/1 -> Subtract/2
  Compare To Constant3/1 -> Gain2/1
  Gain2/1 -> Subtract/3
  Compare To Constant4/1 -> Gain3/1
  Gain3/1 -> Subtract/4
  Compare To Constant5/1 -> Gain4/1
  Gain4/1 -> Subtract/5
  Compare To Constant6/1 -> Gain5/1
  Gain5/1 -> Subtract/6
  Compare To Constant7/1 -> Gain6/1
  Gain6/1 -> Subtract/7
  Compare To Constant8/1 -> Gain7/1
  Gain7/1 -> Subtract/8
  Compare To Constant9/1 -> Gain8/1
  Gain8/1 -> Subtract/9
  Compare To Constant10/1 -> Gain9/1
  Gain9/1 -> Subtract/10
  Compare To Constant11/1 -> Gain10/1
  Gain10/1 -> Subtract/11
  Compare To Constant12/1 -> Gain11/1
  Gain11/1 -> Subtract/12
  Compare To Constant13/1 -> Gain12/1
  Gain12/1 -> Subtract/13
  Compare To Constant14/1 -> Gain13/1
  Gain13/1 -> Subtract/14
  Compare To Constant15/1 -> Gain14/1
  Gain14/1 -> Subtract/15
  Compare To Constant16/1 -> Gain15/1
  Gain15/1 -> Subtract/16
  Compare To Constant17/1 -> Gain16/1
  Gain16/1 -> Subtract/17
  Compare To Constant18/1 -> Gain17/1
  Gain17/1 -> Subtract/18
  Compare To Constant19/1 -> Gain18/1
  Gain18/1 -> Subtract/19
  Compare To Constant20/1 -> Gain19/1
  Gain19/1 -> Subtract/20
  Compare To Constant21/1 -> Gain20/1
  Gain20/1 -> Subtract/21
  Compare To Constant22/1 -> Gain21/1
  Gain21/1 -> Subtract/22
  Compare To Constant23/1 -> Gain22/1
  Gain22/1 -> Subtract/23
  Compare To Constant24/1 -> Gain23/1
  Gain23/1 -> Subtract/24
  Compare To Constant25/1 -> Gain24/1
  Gain24/1 -> Subtract/25
  Compare To Constant26/1 -> Gain25/1
  Gain25/1 -> Subtract/26
  Compare To Constant27/1 -> Gain26/1
  Gain26/1 -> Subtract/27
  Compare To Constant28/1 -> Gain27/1
  Gain27/1 -> Subtract/28
  Compare To Constant29/1 -> Gain28/1
  Gain28/1 -> Subtract/29
  Compare To Constant30/1 -> Gain29/1
  Gain29/1 -> Subtract/30
  Compare To Constant31/1 -> Gain30/1
  Gain30/1 -> Subtract/31
  Compare To Constant32/1 -> Gain31/1
  Gain31/1 -> Subtract/32
  Compare To Constant33/1 -> Gain32/1
  Gain32/1 -> Subtract/33
  Compare To Constant34/1 -> Gain33/1
  Gain33/1 -> Subtract/34
  Compare To Constant35/1 -> Gain34/1
  Gain34/1 -> Subtract/35
  Product1/1 -> Out1/1
  Timer1/1(SineTime_s) -> Product/1
  Logical Operator/1 -> Timer1/Enable
  Detect Change/1 -> Logical Operator1/1
  Logical Operator1/1 -> Logical Operator/2

== system hcu_main_ADASwEPS/EPSS/EPSS/EPSTest/Timer ==
  Enable : EnablePort  StatesWhenEnabling=reset
  C_TASK_1MS_S : Constant  Value=C_TASK_1MS_S
  Sum : Sum  Inputs=|++
  Unit Delay : UnitDelay  SampleTime=-1
  Unit Delay1 : UnitDelay  SampleTime=-1
  SineTime_s : Outport  OutputWhenDisabled=reset  InitialOutput=[0]
  wires:
  Unit Delay1/1 -> Sum/1
  Unit Delay/1 -> Sum/2
  Sum/1 -> SineTime_s/1, Unit Delay/1  "SineTime_s"
  C_TASK_1MS_S/1 -> Unit Delay1/1

== system hcu_main_ADASwEPS/ISP/PassThrough/EPSDegTest/Timer ==
  Enable : EnablePort  StatesWhenEnabling=reset
  C_TASK_1MS_S : Constant  Value=C_TASK_1MS_S
  Sum : Sum  Inputs=|++
  Unit Delay : UnitDelay  SampleTime=-1
  Unit Delay1 : UnitDelay  SampleTime=-1
  SineTime_s : Outport  OutputWhenDisabled=reset  InitialOutput=[0]
  wires:
  Unit Delay1/1 -> Sum/1
  Unit Delay/1 -> Sum/2
  Sum/1 -> SineTime_s/1, Unit Delay/1  "SineTime_s"
  C_TASK_1MS_S/1 -> Unit Delay1/1

== system hcu_main_ADASwEPS/ISP/TqProcessing/TqSensorAZero/Latch ==
  in : Inport
  update : Inport  Port=2
  Delay : Delay  DelayLength=1  InitialCondition=50
  Switch2 : Switch  Criteria=u2 ~= 0  Threshold=0.5
      settings: AttributesFormatString=<Criteria=%<Criteria>>
  out : Outport
  wires:
  Delay/1 -> Switch2/3
  in/1 -> Switch2/1
  Switch2/1 -> out/1, Delay/1
  update/1 -> Switch2/2

== system hcu_main_ADASwEPS/ISP/TqProcessing/TqSensorAZero/Timer ==
  Enable : EnablePort  StatesWhenEnabling=reset
  C_TASK_1MS_S : Constant  Value=C_TASK_1MS_S
  Sum : Sum  Inputs=|++
  Unit Delay : UnitDelay  SampleTime=-1
  Unit Delay1 : UnitDelay  SampleTime=-1
  Time_s : Outport  OutputWhenDisabled=reset  InitialOutput=[0]
  wires:
  Unit Delay1/1 -> Sum/1
  Unit Delay/1 -> Sum/2
  Sum/1 -> Time_s/1, Unit Delay/1  "Time_s"
  C_TASK_1MS_S/1 -> Unit Delay1/1
